simulink model "es2_emg_3"  (R2024a)
settings: Solver=VariableStepAuto  StartTime=0.0  StopTime=30  RelTol=1e-3
libraries: vrlib x1
settings Model: Creator=amisq  LastModifiedBy=amisq

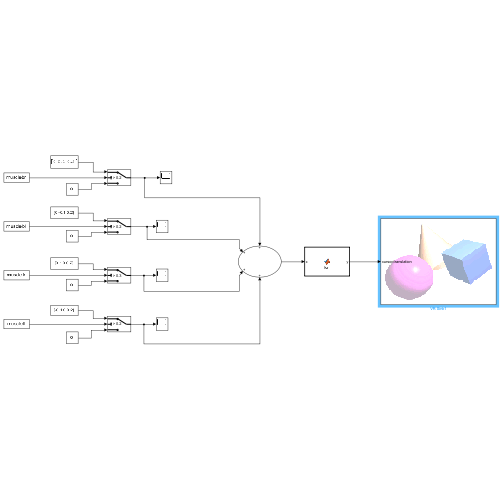
[thumbnail: Simulink's stored preview of the top-level diagram]
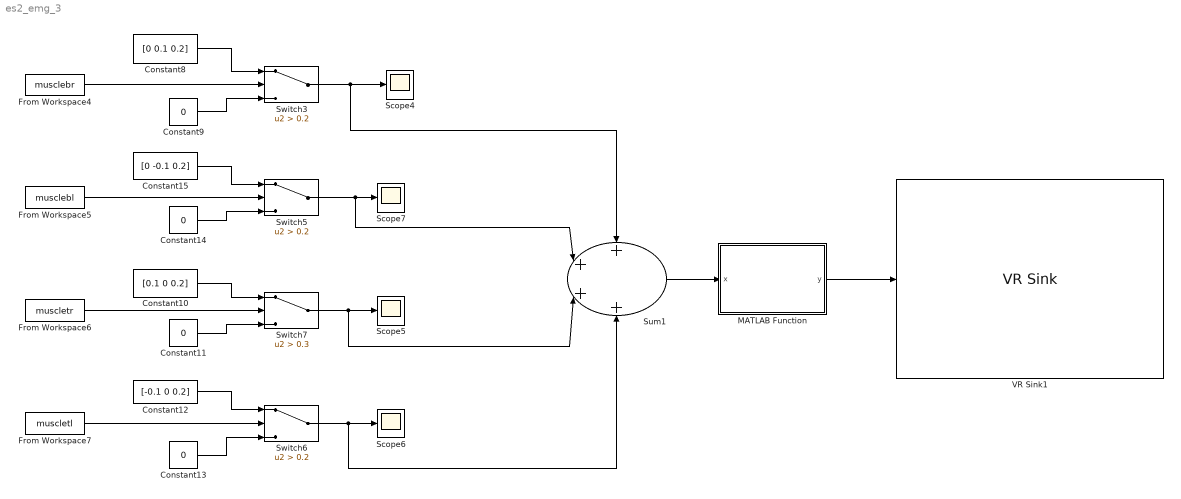
== system es2_emg_3 ==
  Constant10 : Constant  Value=[0.1 0 0.2]
  Constant{9,11,13..14} (4 alike) : Constant  Value=0
  Constant12 : Constant  Value=[-0.1 0 0.2]
  Constant15 : Constant  Value=[0 -0.1 0.2]
  Constant8 : Constant  Value=[0 0.1 0.2]
  From Workspace4 : FromWorkspace  VariableName=musclebr  SampleTime=0.05
  From Workspace5 : FromWorkspace  VariableName=musclebl  SampleTime=0.05
  From Workspace6 : FromWorkspace  VariableName=muscletr  SampleTime=0.05
  From Workspace7 : FromWorkspace  VariableName=muscletl  SampleTime=0.05
  MATLAB Function : MATLAB Function  TreatAsAtomicUnit=on
  Scope{4..7} (4 alike) : Scope
  Sum1 : Sum  Inputs=++++
  Switch3 : Switch  Criteria=u2 > Threshold  Threshold=0.2  SaturateOnIntegerOverflow=off  InputSameDT=off
  Switch5 : Switch  Criteria=u2 > Threshold  Threshold=0.2  SaturateOnIntegerOverflow=off  InputSameDT=off
  Switch6 : Switch  Criteria=u2 > Threshold  Threshold=0.2  SaturateOnIntegerOverflow=off  InputSameDT=off
  Switch7 : Switch  Criteria=u2 > Threshold  Threshold=0.3  SaturateOnIntegerOverflow=off  InputSameDT=off
  VR Sink1 : vrlib/VR Sink  InstantiateOnLoad=on  SampleTime=0.01  ViewEnable=on  RemoteChange=off  RemoteView=off  FieldsWritten=cursor.translation.3.1.1.double  WorldFileName=8_palline_color.wrl  AutoView=off  VideoDimensions=[]  AllowVariableSize=off
  wires:
  Constant11/1 -> Switch7/3
  From Workspace4/1 -> Switch3/2
  Constant13/1 -> Switch6/3
  Constant10/1 -> Switch7/1
  From Workspace6/1 -> Switch7/2
  From Workspace7/1 -> Switch6/2
  Switch7/1 -> Sum1/3, Scope5/1
  Constant15/1 -> Switch5/1
  From Workspace5/1 -> Switch5/2
  Switch6/1 -> Sum1/4, Scope6/1
  Constant14/1 -> Switch5/3
  Switch3/1 -> Sum1/1, Scope4/1
  Switch5/1 -> Sum1/2, Scope7/1
  Constant12/1 -> Switch6/1
  Constant9/1 -> Switch3/3
  Constant8/1 -> Switch3/1
  Sum1/1 -> MATLAB Function/1(x)
  MATLAB Function/1(y) -> VR Sink1/1

== matlab function es2_emg_3/MATLAB Function ==
  data: x input; y output
function y = fcn(x)
      
    if x(1)^2 + x(2)^2 <= 0.1^2
        y = [x(1), x(2), 0.2]; % Mantieni dimensioni fisse
    elseif x(1) > 0.01 && x(2) > 0.01 % caso primo quadrante
        y = [0.07, 0.07, 0.2];
    elseif x(1) < 0.01 && x(2) > 0.01 % caso secondo quadrante
        y = [-0.07, 0.07, 0.2];
    elseif x(1) < 0.01 && x(2) < 0.01 % caso terzo quadrante
        y = [-0.07, -0.07, 0.2];
    elseif x(1) > 0.01 && x(2) < 0.01 % caso quarto quadrante
        y = [0.07, -0.07, 0.2];
    else
        y = [x(1), x(2), 0.2]; % Mantieni dimensioni fisse
    end
end
